simulink model "CLF"  (Simulink 9.1)
settings: Solver=VariableStepAuto  StartTime=0.0  StopTime=40  RelTol=1e-3
libraries: Solver_SF x1, simulink x1
settings Model: Creator=MaoWenJie  LastModifiedBy=MaoWenJie
settings DataIOCC: SaveFormat=Dataset
settings OptimizationCC: LifeSpan=auto
settings DebuggingCC: UnderspecifiedInitializationDetection=Simplified  MergeDetectMultiDrivingBlocksExec=error  SFUnexpectedBacktrackingDiag=error  SFNoUnconditionalDefaultTransitionDiag=error  SFExecutionAtInitializationDiag=warning
settings HardwareCC: ProdBitPerPointer=64  ProdBitPerSizeT=64  ProdBitPerPtrDiffT=64  ProdLargestAtomicFloat=Float  ProdIntDivRoundTo=Zero  ProdEndianess=LittleEndian  ProdWordSize=64  ProdHWDeviceType=Intel->x86-64 (Windows64)
settings ModelReferenceCC: PropagateSignalLabelsOutOfModel=on
settings CodeAppCC: StateflowObjectComments=off
settings GRTTargetCC: TargetLangStandard=C99 (ISO)  CombineOutputUpdateFcns=on  GRTInterface=off
settings ConfigComp: CovMetricSettings=dwe  CovHtmlReporting=off  CovSaveCumulativeToWorkspaceVar=off  CovSaveSingleToWorkspaceVar=off  CovExternalEMLEnable=on

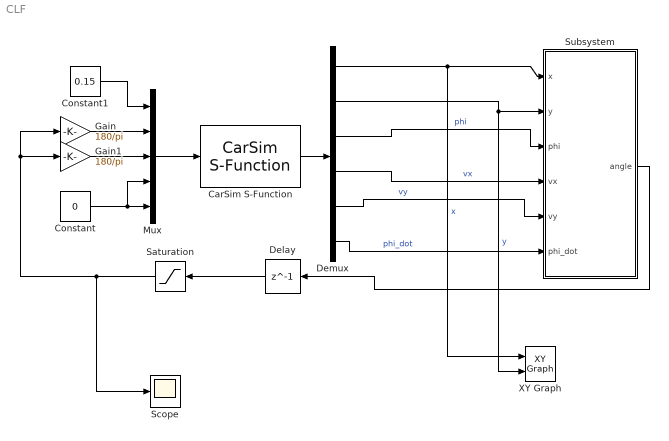
== system CLF ==
  CarSim S-Function : Solver_SF/CarSim S-Function  Priority=1  SIMFILE=simfile.sim
  Constant : Constant  Value=0
  Constant1 : Constant  Value=0.15
  Delay : Delay  DelayLength=1  UseCircularBuffer=on
  Demux : Demux  Outputs=6
  Gain : Gain  Gain=180/pi
  Gain1 : Gain  Gain=180/pi
  Mux : Mux  Inputs=5
  Saturation : Saturate  UpperLimit=1.2  LowerLimit=-1.2
  Scope : Scope
  Subsystem : Subsystem
  XY Graph : simulink/Sinks/XY Graph  xmin=0  xmax=80  ymin=-50  ymax=50  st=-1
  wires:
  Mux/1 -> CarSim S-Function/1
  Demux/6 -> Subsystem/6(phi_dot)  "phi_dot"
  Demux/4 -> Subsystem/4(vx)  "vx"
  CarSim S-Function/1 -> Demux/1
  Demux/3 -> Subsystem/3(phi)  "phi"
  Gain/1 -> Mux/2
  Demux/5 -> Subsystem/5(vy)  "vy"
  Constant1/1 -> Mux/1
  Constant/1 -> Mux/4, Mux/5
  Saturation/1 -> Scope/1, Gain1/1, Gain/1
  Gain1/1 -> Mux/3
  Demux/2 -> XY Graph/2, Subsystem/2(y)  "y"
  Delay/1 -> Saturation/1
  Subsystem/1(angle) -> Delay/1
  Demux/1 -> XY Graph/1, Subsystem/1(x)  "x"

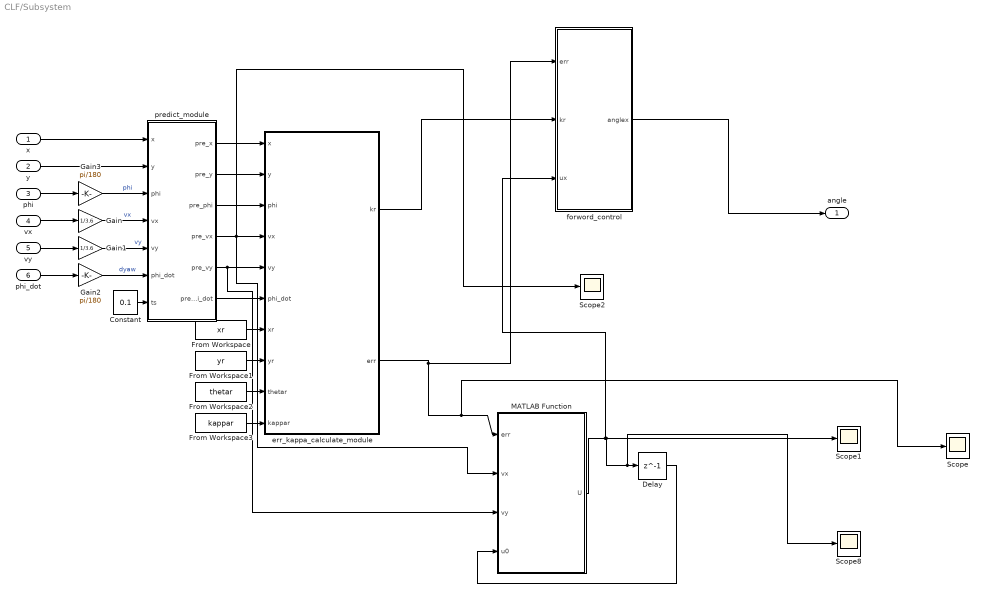
== system CLF/Subsystem ==
  x : Inport
  y : Inport  Port=2
  phi : Inport  Port=3
  vx : Inport  Port=4
  vy : Inport  Port=5
  phi_dot : Inport  Port=6
  Constant : Constant  Value=0.1
  Delay : Delay  DelayLength=1  InitialCondition=0
  From Workspace : FromWorkspace  VariableName=xr  SampleTime=0
  From Workspace1 : FromWorkspace  VariableName=yr  SampleTime=0
  From Workspace2 : FromWorkspace  VariableName=thetar  SampleTime=0
  From Workspace3 : FromWorkspace  VariableName=kappar  SampleTime=0
  Gain : Gain  Gain=1/3.6
  Gain1 : Gain  Gain=1/3.6
  Gain2 : Gain  Gain=pi/180
  Gain3 : Gain  Gain=pi/180
  MATLAB Function : MATLAB Function  InitFcn=u0 = zeros(1,1);err = [0;0;0;0];vx = 0;vy=0;  TreatAsAtomicUnit=on
  Scope{,1..2,8} (4 alike) : Scope
  err_kappa_calculate_module : MATLAB Function  TreatAsAtomicUnit=on
  forword_control : MATLAB Function  TreatAsAtomicUnit=on
  predict_module : MATLAB Function  TreatAsAtomicUnit=on
  angle : Outport
  wires:
  Gain1/1 -> predict_module/5(vy)  "vy"
  x/1 -> predict_module/1(x)
  phi_dot/1 -> Gain2/1
  predict_module/2(pre_y) -> err_kappa_calculate_module/2(y)
  vx/1 -> Gain/1
  predict_module/4(pre_vx) -> Scope2/1, MATLAB Function/2(vx), err_kappa_calculate_module/4(vx)
  Gain2/1 -> predict_module/6(phi_dot)  "dyaw"
  phi/1 -> Gain3/1
  From Workspace2/1 -> err_kappa_calculate_module/9(thetar)
  Gain/1 -> predict_module/4(vx)  "vx"
  y/1 -> predict_module/2(y)
  Gain3/1 -> predict_module/3(phi)  "phi"
  From Workspace3/1 -> err_kappa_calculate_module/10(kappar)
  Constant/1 -> predict_module/7(ts)
  From Workspace1/1 -> err_kappa_calculate_module/8(yr)
  predict_module/1(pre_x) -> err_kappa_calculate_module/1(x)
  predict_module/5(pre_vy) -> MATLAB Function/3(vy), err_kappa_calculate_module/5(vy)
  vy/1 -> Gain1/1
  From Workspace/1 -> err_kappa_calculate_module/7(xr)
  predict_module/6(pre_phi_dot) -> err_kappa_calculate_module/6(phi_dot)
  predict_module/3(pre_phi) -> err_kappa_calculate_module/3(phi)
  err_kappa_calculate_module/2(err) -> forword_control/1(err), Scope/1, MATLAB Function/1(err)
  err_kappa_calculate_module/1(kr) -> forword_control/2(kr)
  forword_control/1(anglex) -> angle/1
  MATLAB Function/1(U) -> Scope1/1, Scope8/1, Delay/1, forword_control/3(ux)
  Delay/1 -> MATLAB Function/4(u0)

== matlab function Subsystem/err_kappa_calculate_module ==
  data: x input double; kr output double; y input double; phi input double; vx input double; vy input double; phi_dot input double; xr input double; yr input double; thetar input double; kappar input double; err output double
function [kr,err] = fcn(x,y,phi,vx,vy,phi_dot,xr,yr,thetar,kappar)
    n=length(xr);
    d_min=(x-xr(1))^2+(y-yr(1))^2;
    min=1;
    for i=1:n
        d=(x-xr(i))^2+(y-yr(i))^2;
        if d<d_min
            d_min=d;
            min=i;
        end
    end
    dmin=min;
    tor=[cos(thetar(dmin));sin(thetar(dmin))];
    nor=[-sin(thetar(dmin));cos(thetar(dmin))];
    d_err=[x-xr(dmin);y-yr(dmin)];
    ed=nor'*d_err;
    es=tor'*d_err;
    %projection_point_thetar=thetar(dmin);%apollo
    projection_point_thetar=thetar(dmin)+kappar(dmin)*es;
    ed_dot=vy*cos(phi-projection_point_thetar)+vx*sin(phi-projection_point_thetar);
    %%%%%%%%%
    ephi=sin(phi-projection_point_thetar);
    %%%%%%%%%
    s_dot=vx*cos(phi-projection_point_thetar)-vy*sin(phi-projection_point_thetar);
    s_dot=s_dot/(1-kappar(dmin)*ed);
    ephi_dot=phi_dot-kappar(dmin)*s_dot;
    kr=kappar(dmin);
    err=[ed;ed_dot;ephi;ephi_dot];
    
    
    
    
    
    
    
    
    
    
    
    


end

== matlab function Subsystem/predict_module ==
  data: x input double; pre_x output double; y input double; phi input double; vx input double; vy input double; phi_dot input double; ts input double; pre_y output double; pre_phi output double; pre_vx output double; pre_vy output double; pre_phi_dot output double
function [pre_x,pre_y,pre_phi,pre_vx,pre_vy,pre_phi_dot] = fcn(x,y,phi,vx,vy,phi_dot,ts)
    pre_x=x+vx*ts*cos(phi)-vy*ts*sin(phi);
    pre_y=y+vy*ts*cos(phi)+vx*ts*sin(phi);
    pre_phi=phi+phi_dot*ts;
    pre_vx=vx;
    pre_vy=vy;
    pre_phi_dot=phi_dot;
end

== matlab function Subsystem/forword_control ==
  data: err input double; anglex output double; kr input double; ux input double
function anglex = fcn(err, kr,ux)
    a=1.015;
    b=2.910-1.015;
    anglex = atan((kr*cos(err(3)*(a+b)))/(1-err(1)*kr)+ux);
end

== matlab function Subsystem/MATLAB Function ==
  data: err input double; vx input double; vy input double; U output double; u0 input double
function U   = ...
    CLF_control(err,vx,vy,u0) 
coder.extrinsic('dlqr');
coder.extrinsic('optimoptions');
coder.extrinsic('quadprog');
a=1.015;
b=2.910-1.015;
v = sqrt(vx^2+vy^2);
x = [err(1);err(3)];
fx = [v*sin(x(2));0];
gx = [0;v/(a+b)];
V = x'*x/2;
dVx = x;
LfV = dVx'*fx;
LgV = dVx'*gx;
gamma = 2;%0.5
h = -v*x(1)*sin(x(2))-gamma*x(1)^2/2;
Lfh = -v^2*sin(x(2))^2-gamma*x(1)*v*sin(x(2));
Lgh = -v^2*x(1)*cos(x(2))/(a+b);
alpha = 10;%10
%----------------avoid obstacle-------------------------------
% dsafe = 1.955;
% d = (xv-xo)^2+(yv-yo)^2-dsafe^2;
% dotd = 2*(xv-xo)*v*cos(theta)+2*(yv-yo)*v*sin(theta);
% %dotd = dotd*0.4;
% B =  d + dotd*0.4;%exp(-0.1*d+0.1)
% LfB = dotd+2*v^2*0.4;
% LgB = (-2*(xv-xo)*v*sin(theta)/(a+b)+2*(yv-yo)*v*cos(theta)/(a+b))*0.4;
%-------------------------------------------------------------
% u = 0;
% u = sdpvar(1,1); % 决策变量
Umin = [-tan(1.2);0];%0.58
Umax = [tan(1.2);200];
% Constraints = [LfV + LgV*u + gamma*V <= 0];% CLF约束
% Constraints = [Constraints; Umin<=u<=Umax];
% Objective = 0.5*u'*u;
% Options = sdpsettings('verbose',0,'solver','quadprog');
% sol.yalmipversion = '20210331';
% sol.matlabversion = '9.4.0.813654 (R2018a)';
% sol.yalmiptime = 0.0431;
% sol.solvertime = 0.0029;
% sol.info = 'Successfully solved (QUADPROG)';
% sol.problem = 0;
% sol = solvesdp([LfV + LgV*u + gamma*V <= 0;Umin<=u<=Umax],Objective, Options);
% U = 0;
% if sol.problem == 0
%     U = double(value(u));
% else
%     U = u0;
% end
% l = Umax;
% a = LgV;
% b = LfV+gamma*V;
% if(b-abs(a*l)>0)
%     U = u0;
% else
%     if(b<=0)
%     U = 0;
%     else
%     U = -b/a;
%     end
% end
%% 开始求解过程
H = zeros(2,2);
p = 0.1;
H(1,1) = 0.5;
H(2,2) = 0.5*p;
U = 0;
%delta = 0;
exitflag = 0.5;
X0=zeros(2,1);
A = [-Lgh -1];
AV = [LgV -1];
%----------------avoid obstacle-------------------------------
% alpha_avoid = 5;
% A_avoid = [-Lgh -1;
%            -LgB 0];
% b_avoid = [alpha*h+Lfh;
%            alpha_avoid*B+LfB];
%-------------------------------------------------------------
options = optimoptions('quadprog','Display','iter','MaxIterations',100,'TolFun',1e-16);
%[X,fval,exitflag]=quadprog(H,[],AV,-LfV-gamma*V,[],[],Umin,Umax,X0,options);
[X,fval,exitflag]=quadprog(H,[],A,Lfh+alpha*h,[],[],Umin,Umax,X0,options);
% if LgB>10
%     [X,fval,exitflag]=quadprog(H,[],A_avoid,b_avoid,[],[],Umin,Umax,X0,options);
% else
%     if x(1)>0
%     Umin = 0.02*d;
%     Umax = 9999;
%     else
%     Umin = -9999;
%     Umax = -0.02*d;
%     end
%     [X,fval,exitflag]=quadprog(H,[],A_avoid,b_avoid,[],[],Umin,Umax,X0,options);
% end
%% 计算输出
if exitflag==-2
U = u0;
else
U = X(1);
end
a = Lgh;
b = Lfh+alpha*h;
end
